simulink subsystem "rss_motor_model"  (R2023a)
settings: Solver=VariableStepAuto  StartTime=0.0  StopTime=10.0  RelTol=1e-3
undefined symbols (not defined in the file): Cdbl_indPhIndcPeakVal, Cdbl_psiPermMagFlxPeakVal, Cdbl_resPhRstnPeakVal, cstPermMagTempCoef, cstPhsRsntTempCoef, Gu16_indDaxIndc_C, Gu16_indQaxIndc_C, Gu16_psiPermMagFlx_C, Gu16_resPhRstn_C, Gu8_numPPNum_C, parAmbPermMagFlux_u16p22b0, parAmbPhsRsnt_u16p20b0, parDirIndc_u16p29b0, parGmrSensAngErrInpData, parGmrSensAngErrLktData, parMotRtrInrt, parMotTorsViscDamp, parPermMagTempCoef_s16p23b0, parPhsRsntTempCoef_s16p23b0, parPolePairNum_u8n0b0, parQdrtIndc_u16p29b0
libraries: mcbcontrolslib x4, MERMASS11MSEREF x3, eeTransforms x2, EMPSMDQ301MSEREF x2, lib_park_transform x2, EMPSMD3E01MSEREF x1, autolibpmsminterior x1, autolibsharedcoupling x1, simulink x1
settings Model: Creator=CAV2OFO  LastModifiedBy=xiaoqiang.yuan
settings SolverCC: AlgebraicLoopSolver=TrustRegion
settings OptimizationCC: ReuseModelBlockBuffer=off
settings DebuggingCC: UnconnectedInputMsg=warning  UnconnectedOutputMsg=warning  UnconnectedLineMsg=warning
settings ModelReferenceCC: EnableRefExpFcnMdlSchedulingChecks=on
settings RTWCC: DLArmComputeVersion=19.05

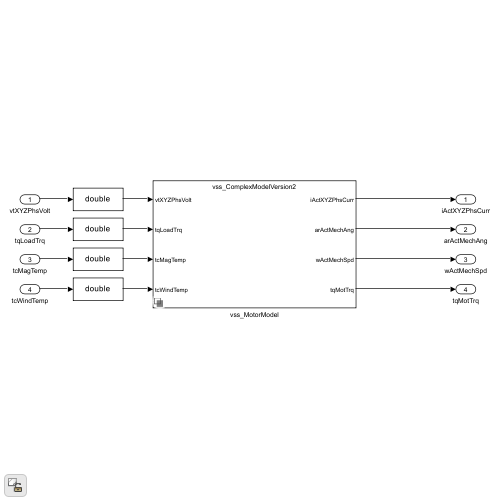
[thumbnail: Simulink's stored preview of the top-level diagram]
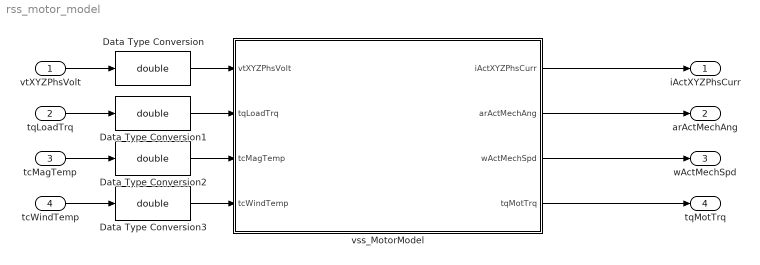
== system rss_motor_model ==
  vtXYZPhsVolt : Inport
  tqLoadTrq : Inport  Port=2
  tcMagTemp : Inport  Port=3
  tcWindTemp : Inport  Port=4
  Data Type Conversion{,1..3} (4 alike) : DataTypeConversion  OutDataTypeStr=double  SaturateOnIntegerOverflow=off  RndMeth=Floor
  vss_MotorModel : Subsystem  Variant=on  VariantControlMode=label  LabelModeActiveChoice=parCompMdlVrs2Lbl
  iActXYZPhsCurr : Outport
  arActMechAng : Outport  Port=2
  wActMechSpd : Outport  Port=3
  tqMotTrq : Outport  Port=4
  wires:
  vss_MotorModel/3(wActMechSpd) -> wActMechSpd/1
  vss_MotorModel/1(iActXYZPhsCurr) -> iActXYZPhsCurr/1
  vss_MotorModel/2(arActMechAng) -> arActMechAng/1
  tqLoadTrq/1 -> Data Type Conversion1/1
  vss_MotorModel/4(tqMotTrq) -> tqMotTrq/1
  vtXYZPhsVolt/1 -> Data Type Conversion/1
  tcMagTemp/1 -> Data Type Conversion2/1
  tcWindTemp/1 -> Data Type Conversion3/1
  Data Type Conversion/1 -> vss_MotorModel/1(vtXYZPhsVolt)
  Data Type Conversion1/1 -> vss_MotorModel/2(tqLoadTrq)
  Data Type Conversion3/1 -> vss_MotorModel/4(tcWindTemp)
  Data Type Conversion2/1 -> vss_MotorModel/3(tcMagTemp)

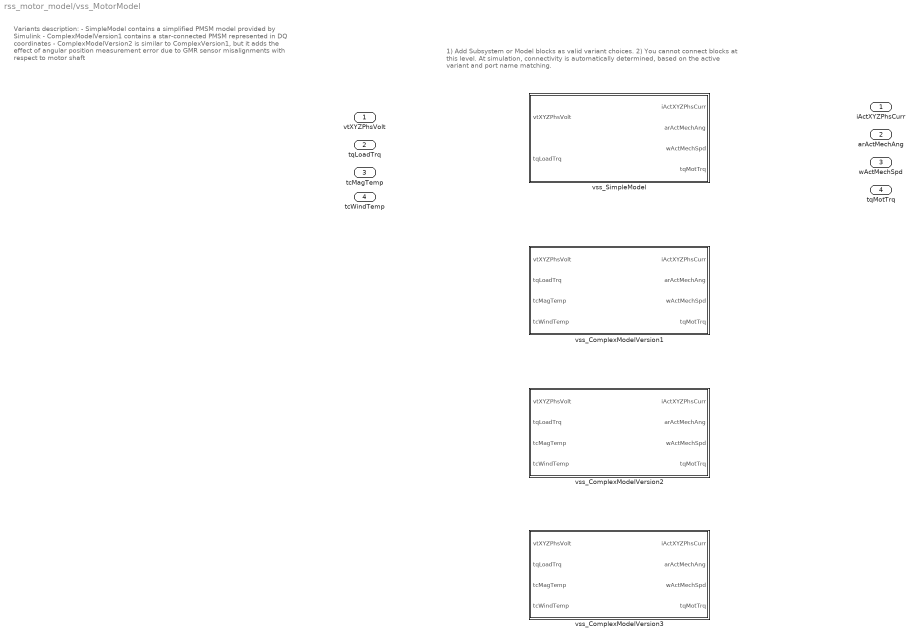
== system rss_motor_model/vss_MotorModel ==
  note: 1) Add Subsystem or Model blocks as valid variant choices.
      | 2) You cannot connect blocks at this level. At simulation, connectivity is automatically
      | determined, based on the active variant and port name matching.
  note: Variants description:
      | - SimpleModel contains a simplified PMSM model provided by Simulink
      | - ComplexModelVersion1 contains a star-connected PMSM represented
      | in DQ coordinates
      | - ComplexModelVersion2 is similar to ComplexVersion1, but it adds the
      | effect of angular position measurement error due to GMR sensor misalignments
      | with respect to motor shaft
  vtXYZPhsVolt : Inport
  tqLoadTrq : Inport  Port=2
  tcMagTemp : Inport  Port=3
  tcWindTemp : Inport  Port=4
  vss_ComplexModelVersion1 : Subsystem  VariantControl=parCompMdlVrs1Lbl
  vss_ComplexModelVersion2 : Subsystem  VariantControl=parCompMdlVrs2Lbl
  vss_ComplexModelVersion3 : Subsystem  VariantControl=Choice
  vss_SimpleModel : Subsystem  VariantControl=parSmplMdlLbl
  iActXYZPhsCurr : Outport
  arActMechAng : Outport  Port=2
  wActMechSpd : Outport  Port=3
  tqMotTrq : Outport  Port=4

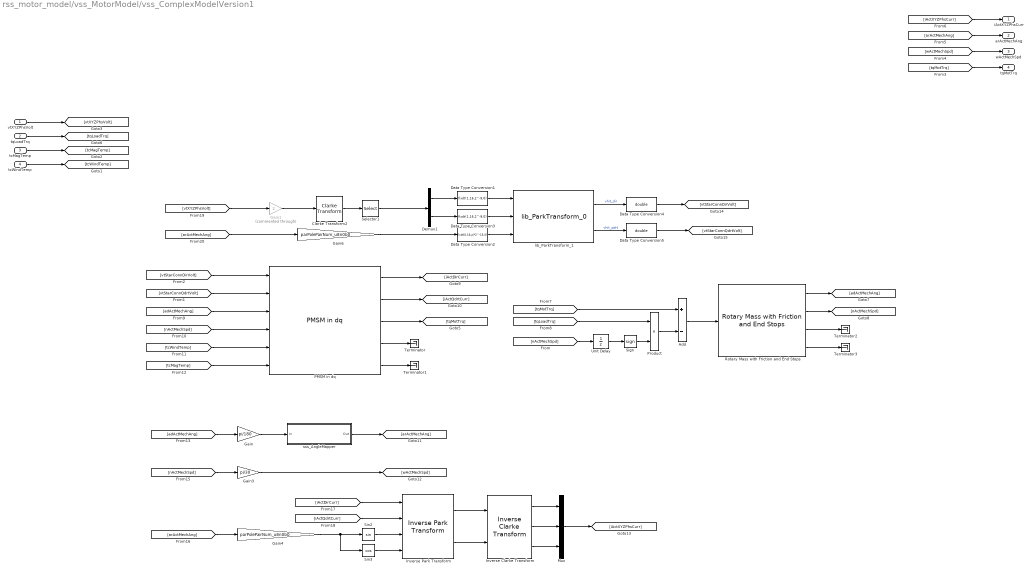
== system rss_motor_model/vss_MotorModel/vss_ComplexModelVersion1 ==
  vtXYZPhsVolt : Inport
  tqLoadTrq : Inport  Port=2
  tcMagTemp : Inport  Port=3
  tcWindTemp : Inport  Port=4
  Add : Sum  Inputs=+-
  Clarke Transform2 : eeTransforms/Clarke Transform  PowerInvariant=off
  Data Type Conversion1 : DataTypeConversion  OutDataTypeStr=fixdt(1,16,2^-9,0)  SaturateOnIntegerOverflow=off  RndMeth=Floor
  Data Type Conversion2 : DataTypeConversion  OutDataTypeStr=fixdt(0,16,pi*2^-15,0)  SaturateOnIntegerOverflow=off  RndMeth=Floor
  Data Type Conversion3 : DataTypeConversion  OutDataTypeStr=fixdt(1,16,2^-9,0)  SaturateOnIntegerOverflow=off  RndMeth=Floor
  Data Type Conversion4 : DataTypeConversion  OutDataTypeStr=double  SaturateOnIntegerOverflow=off  RndMeth=Floor
  Data Type Conversion5 : DataTypeConversion  OutDataTypeStr=double  SaturateOnIntegerOverflow=off  RndMeth=Floor
  Demux1 : Demux  Outputs=2
  Gain : Gain  Gain=pi/180
  Gain1 : Gain  Commented=through  Gain=2
  Gain3 : Gain  Gain=pi/30
  Gain4 : Gain  Gain=parPolePairNum_u8n0b0  OutDataTypeStr=double
  Gain6 : Gain  Gain=parPolePairNum_u8n0b0  OutDataTypeStr=double
  Inverse Clarke Transform : mcbcontrolslib/Inverse Clarke Transform  PhaseInput=Two inputs  EnPowerInv=off
  Inverse Park Transform : mcbcontrolslib/Inverse Park Transform  PhaseInput=Two inputs  AxisAlignment=D-axis  ThetaInput=Sine and Cosine electrical position  AngleInput=Per-unit  N_points=1024
  Mux : Mux  Inputs=3
  PMSM in dq : EMPSMDQ301MSEREF/PMSM in dq  Tag=EMPSMDQ301MSEREF  N=double(parPolePairNum_u8n0b0)  R20=double(parAmbPhsRsnt_u16p20b0)  Ld=double(parDirIndc_u16p29b0)  Lq=double(parQdrtIndc_u16p29b0)  Km20=double(parAmbPermMagFlux_u16p22b0)  Acog=0  Ncog=0  alpha=double(parPhsRsntTempCoef_s16p23b0)  alphamag=double(parPermMagTempCoef_s16p23b0)  xIdinit=0  xIqinit=0
      settings: AttributesFormatString=<%<Tag>>
  Product : Product
  Rotary Mass with Friction and End Stops : MERMASS11MSEREF/Rotary Mass with Friction and End Stops  Tag=MERMASS11MSEREF  J=double(parMotRtrInrt)  dvisc=double(parMotTorsViscDamp)*pi/30  frictionmode=no friction  epsn=0.001  tauinv=1000  TStick=1  TCoulomb=0.9  nStri=0.01  endstopmode=no end stop  phimin=-1e6  phimax=1e6  cstop=1e6  kimpact=0.5  phiinit=0  nRPMinit=0
      settings: AttributesFormatString=<%<Tag>>
  Selector1 : Selector  InputPortWidth=3  IndexOptions=Index vector (dialog)  Indices=[1 2]  OutputSizes=1
  Sign : Signum
  Sin2 : Trigonometry
  Sin3 : Trigonometry  Operator=cos
  Terminator{,1..3} (4 alike) : Terminator
  Unit Delay : UnitDelay  SampleTime=-1  HasFrameUpgradeWarning=on
  lib_ParkTransform_1 : lib_park_transform/lib_ParkTransform_0  VariantControl=ClarkTransf_MIL_flo  lb_parSelRotFrmeAxis=d-axis
  sss_AngleMapper : Subsystem
  iActXYZPhsCurr : Outport
  arActMechAng : Outport  Port=2
  wActMechSpd : Outport  Port=3
  tqMotTrq : Outport  Port=4
  wires:
  [arActMechAng] -> arActMechAng/1
  [tqLoadTrq] -> Product/1
  Unit Delay/1 -> Sign/1
  Sign/1 -> Product/2
  Product/1 -> Add/2
  [nActMechSpd] -> Unit Delay/1
  Gain1/1 -> Clarke Transform2/1
  Gain6/1 -> Data Type Conversion2/1
  Data Type Conversion5/1 -> [vtStarConnQdrtVolt]
  Clarke Transform2/1 -> Selector1/1
  lib_ParkTransform_1/1 -> Data Type Conversion4/1  "vhit_dir"
  [vtXYZPhsVolt] -> Gain1/1
  [arActMechAng] -> Gain6/1
  Data Type Conversion3/1 -> lib_ParkTransform_1/2
  Data Type Conversion1/1 -> lib_ParkTransform_1/1
  Data Type Conversion2/1 -> lib_ParkTransform_1/3
  Demux1/1 -> Data Type Conversion1/1
  Selector1/1 -> Demux1/1
  Demux1/2 -> Data Type Conversion3/1
  Data Type Conversion4/1 -> [vtStarConnDirVolt]
  lib_ParkTransform_1/2 -> Data Type Conversion5/1  "vhit_qdrt"
  Inverse Clarke Transform/3 -> Mux/3
  tcWindTemp/1 -> [tcWindTemp]
  [tcWindTemp] -> PMSM in dq/5
  Gain4/1 -> Sin2/1, Sin3/1
  Mux/1 -> [iActXYZPhsCurr]
  Inverse Park Transform/2 -> Inverse Clarke Transform/2
  Rotary Mass with Friction and End Stops/1 -> [adActMechAng]
  PMSM in dq/4 -> Terminator/1
  [arActMechAng] -> Gain4/1
  Rotary Mass with Friction and End Stops/4 -> Terminator3/1
  tqLoadTrq/1 -> [tqLoadTrq]
  [tqMotTrq] -> tqMotTrq/1
  vtXYZPhsVolt/1 -> [vtXYZPhsVolt]
  PMSM in dq/2 -> [iActQdrtCurr]
  [vtStarConnDirVolt] -> PMSM in dq/1
  [nActMechSpd] -> Gain3/1
  [iActDirCurr] -> Inverse Park Transform/1
  [iActQdrtCurr] -> Inverse Park Transform/2
  [adActMechAng] -> PMSM in dq/3
  Rotary Mass with Friction and End Stops/3 -> Terminator2/1
  [tcMagTemp] -> PMSM in dq/6
  Inverse Clarke Transform/1 -> Mux/1
  Inverse Park Transform/1 -> Inverse Clarke Transform/1
  PMSM in dq/5 -> Terminator1/1
  Gain3/1 -> [wActMechSpd]
  [tqMotTrq] -> Add/1
  [nActMechSpd] -> PMSM in dq/4
  sss_AngleMapper/1(Out) -> [arActMechAng]
  [vtStarConnQdrtVolt] -> PMSM in dq/2
  [wActMechSpd] -> wActMechSpd/1
  [iActXYZPhsCurr] -> iActXYZPhsCurr/1
  tcMagTemp/1 -> [tcMagTemp]
  PMSM in dq/3 -> [tqMotTrq]
  [adActMechAng] -> Gain/1
  Inverse Clarke Transform/2 -> Mux/2
  Add/1 -> Rotary Mass with Friction and End Stops/1
  Gain/1 -> sss_AngleMapper/1(In)
  Sin3/1 -> Inverse Park Transform/4
  Sin2/1 -> Inverse Park Transform/3
  PMSM in dq/1 -> [iActDirCurr]
  Rotary Mass with Friction and End Stops/2 -> [nActMechSpd]

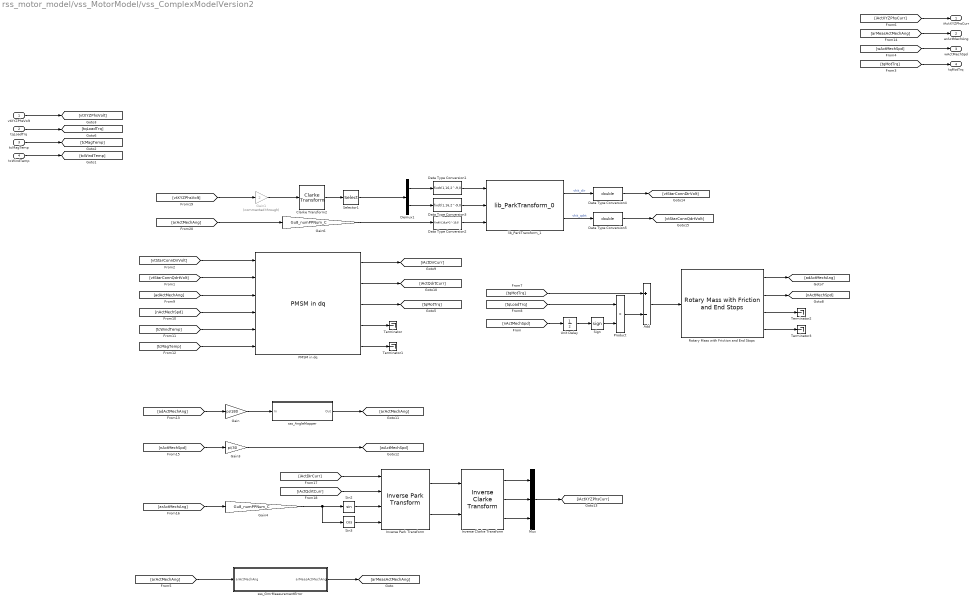
== system rss_motor_model/vss_MotorModel/vss_ComplexModelVersion2 ==
  vtXYZPhsVolt : Inport
  tqLoadTrq : Inport  Port=2
  tcMagTemp : Inport  Port=3
  tcWindTemp : Inport  Port=4
  Add : Sum  Inputs=+-
  Clarke Transform2 : eeTransforms/Clarke Transform  PowerInvariant=off
  Data Type Conversion1 : DataTypeConversion  OutDataTypeStr=fixdt(1,16,2^-9,0)  SaturateOnIntegerOverflow=off  RndMeth=Floor
  Data Type Conversion2 : DataTypeConversion  OutDataTypeStr=fixdt(0,16,pi*2^-15,0)  SaturateOnIntegerOverflow=off  RndMeth=Floor
  Data Type Conversion3 : DataTypeConversion  OutDataTypeStr=fixdt(1,16,2^-9,0)  SaturateOnIntegerOverflow=off  RndMeth=Floor
  Data Type Conversion4 : DataTypeConversion  OutDataTypeStr=double  SaturateOnIntegerOverflow=off  RndMeth=Floor
  Data Type Conversion5 : DataTypeConversion  OutDataTypeStr=double  SaturateOnIntegerOverflow=off  RndMeth=Floor
  Demux1 : Demux  Outputs=2
  Gain : Gain  Gain=pi/180
  Gain1 : Gain  Commented=through  Gain=2
  Gain3 : Gain  Gain=pi/30
  Gain4 : Gain  Gain=Gu8_numPPNum_C  OutDataTypeStr=double
  Gain6 : Gain  Gain=Gu8_numPPNum_C  OutDataTypeStr=double
  Inverse Clarke Transform : mcbcontrolslib/Inverse Clarke Transform
  Inverse Park Transform : mcbcontrolslib/Inverse Park Transform  AxisAlignment=D-axis
  Mux : Mux  Inputs=3
  PMSM in dq : EMPSMDQ301MSEREF/PMSM in dq  Tag=EMPSMDQ301MSEREF  N=double(Gu8_numPPNum_C)  R20=double(Gu16_resPhRstn_C*Cdbl_resPhRstnPeakVal)  Ld=double(Gu16_indDaxIndc_C*Cdbl_indPhIndcPeakVal)  Lq=double(Gu16_indQaxIndc_C*Cdbl_indPhIndcPeakVal)  Km20=double(Gu16_psiPermMagFlx_C*Cdbl_psiPermMagFlxPeakVal)  Acog=0  Ncog=0  alpha=double(cstPhsRsntTempCoef)  alphamag=double(cstPermMagTempCoef)  xIdinit=0  xIqinit=0
      settings: AttributesFormatString=<%<Tag>>
  Product : Product
  Rotary Mass with Friction and End Stops : MERMASS11MSEREF/Rotary Mass with Friction and End Stops  Tag=MERMASS11MSEREF  J=double(parMotRtrInrt)  dvisc=double(parMotTorsViscDamp)*pi/30  frictionmode=no friction  epsn=0.001  tauinv=1000  TStick=1  TCoulomb=0.9  nStri=0.01  endstopmode=no end stop  phimin=-1e6  phimax=1e6  cstop=1e6  kimpact=0.5  phiinit=rand*360  nRPMinit=0
      settings: AttributesFormatString=<%<Tag>>
  Selector1 : Selector  InputPortWidth=3  IndexOptions=Index vector (dialog)  Indices=[1 2]  OutputSizes=1
  Sign : Signum
  Sin2 : Trigonometry
  Sin3 : Trigonometry  Operator=cos
  Terminator{,1..3} (4 alike) : Terminator
  Unit Delay : UnitDelay  SampleTime=-1  HasFrameUpgradeWarning=on
  lib_ParkTransform_1 : lib_park_transform/lib_ParkTransform_0  VariantControl=ClarkTransf_MIL_flo  lb_parSelRotFrmeAxis=d-axis
  sss_AngleMapper : Subsystem
  sss_GmrMeasurementError : Subsystem
  iActXYZPhsCurr : Outport
  arActMechAng : Outport  Port=2
  wActMechSpd : Outport  Port=3
  tqMotTrq : Outport  Port=4
  wires:
  sss_GmrMeasurementError/1(arMeasActMechAng) -> [arMeasActMechAng]
  [arMeasActMechAng] -> arActMechAng/1
  [arActMechAng] -> sss_GmrMeasurementError/1(arActMechAng)
  [tqLoadTrq] -> Product/1
  Unit Delay/1 -> Sign/1
  Sign/1 -> Product/2
  Product/1 -> Add/2
  [nActMechSpd] -> Unit Delay/1
  Gain1/1 -> Clarke Transform2/1
  Gain6/1 -> Data Type Conversion2/1
  Data Type Conversion5/1 -> [vtStarConnQdrtVolt]
  Clarke Transform2/1 -> Selector1/1
  lib_ParkTransform_1/1 -> Data Type Conversion4/1  "vhit_dir"
  [vtXYZPhsVolt] -> Gain1/1
  [arActMechAng] -> Gain6/1
  Data Type Conversion3/1 -> lib_ParkTransform_1/2
  Data Type Conversion1/1 -> lib_ParkTransform_1/1
  Data Type Conversion2/1 -> lib_ParkTransform_1/3
  Demux1/1 -> Data Type Conversion1/1
  Selector1/1 -> Demux1/1
  Demux1/2 -> Data Type Conversion3/1
  Data Type Conversion4/1 -> [vtStarConnDirVolt]
  lib_ParkTransform_1/2 -> Data Type Conversion5/1  "vhit_qdrt"
  Inverse Clarke Transform/3 -> Mux/3
  tcWindTemp/1 -> [tcWindTemp]
  [tcWindTemp] -> PMSM in dq/5
  Gain4/1 -> Sin2/1, Sin3/1
  Mux/1 -> [iActXYZPhsCurr]
  Inverse Park Transform/2 -> Inverse Clarke Transform/2
  Rotary Mass with Friction and End Stops/1 -> [adActMechAng]
  PMSM in dq/4 -> Terminator/1
  [arActMechAng] -> Gain4/1
  Rotary Mass with Friction and End Stops/4 -> Terminator3/1
  tqLoadTrq/1 -> [tqLoadTrq]
  [tqMotTrq] -> tqMotTrq/1
  vtXYZPhsVolt/1 -> [vtXYZPhsVolt]
  PMSM in dq/2 -> [iActQdrtCurr]
  [vtStarConnDirVolt] -> PMSM in dq/1
  [nActMechSpd] -> Gain3/1
  [iActDirCurr] -> Inverse Park Transform/1
  [iActQdrtCurr] -> Inverse Park Transform/2
  [adActMechAng] -> PMSM in dq/3
  Rotary Mass with Friction and End Stops/3 -> Terminator2/1
  [tcMagTemp] -> PMSM in dq/6
  Inverse Clarke Transform/1 -> Mux/1
  Inverse Park Transform/1 -> Inverse Clarke Transform/1
  PMSM in dq/5 -> Terminator1/1
  Gain3/1 -> [wActMechSpd]
  [tqMotTrq] -> Add/1
  [nActMechSpd] -> PMSM in dq/4
  sss_AngleMapper/1(Out) -> [arActMechAng]
  [vtStarConnQdrtVolt] -> PMSM in dq/2
  [wActMechSpd] -> wActMechSpd/1
  [iActXYZPhsCurr] -> iActXYZPhsCurr/1
  tcMagTemp/1 -> [tcMagTemp]
  PMSM in dq/3 -> [tqMotTrq]
  [adActMechAng] -> Gain/1
  Inverse Clarke Transform/2 -> Mux/2
  Add/1 -> Rotary Mass with Friction and End Stops/1
  Gain/1 -> sss_AngleMapper/1(In)
  Sin3/1 -> Inverse Park Transform/4
  Sin2/1 -> Inverse Park Transform/3
  PMSM in dq/1 -> [iActDirCurr]
  Rotary Mass with Friction and End Stops/2 -> [nActMechSpd]

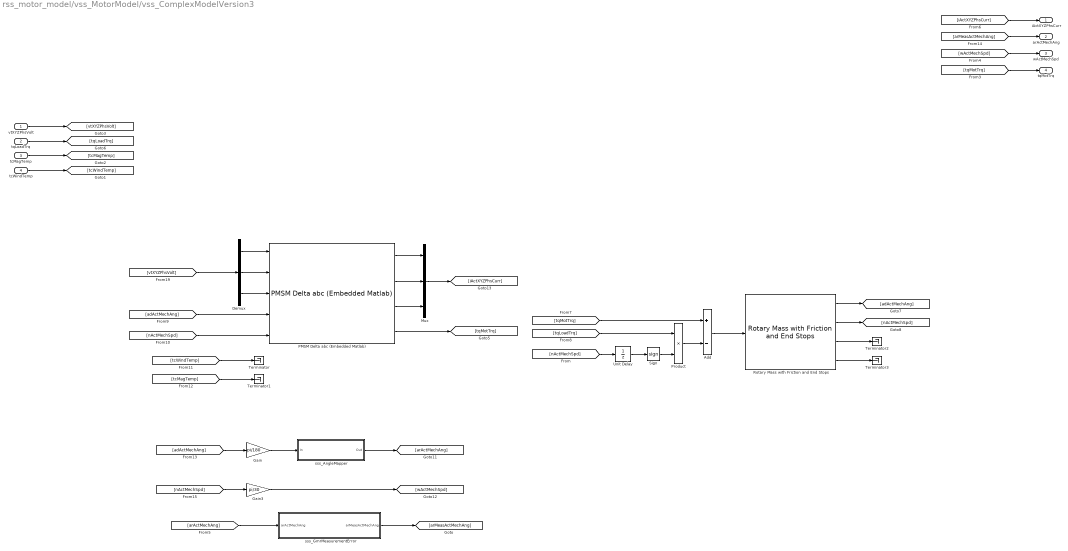
== system rss_motor_model/vss_MotorModel/vss_ComplexModelVersion3 ==
  vtXYZPhsVolt : Inport
  tqLoadTrq : Inport  Port=2
  tcMagTemp : Inport  Port=3
  tcWindTemp : Inport  Port=4
  Add : Sum  Inputs=+-
  Demux : Demux  Outputs=3
  Gain : Gain  Gain=pi/180
  Gain3 : Gain  Gain=pi/30
  Mux : Mux  Inputs=3
  PMSM Delta abc (Embedded Matlab) : EMPSMD3E01MSEREF/PMSM Delta abc (Embedded Matlab)  Tag=EMPSMD3E01MSEREF  N=double(parPolePairNum_u8n0b0)  r_m=double(parAmbPhsRsnt_u16p20b0)*3/2  l=[(double(parDirIndc_u16p29b0)+double(parQdrtIndc_u16p29b0))/2 0 (double(parDirIndc_u16p29b0)-double(parQdrtIndc_u16p29b0)) 0 0]*3/2  m=[0 0 0 0 0]  Km=double(parAmbPermMagFlux_u16p22b0)  a357=[0]  xIainit=0.0  xIbinit=0.0  xIcinit=0.0
      settings: AttributesFormatString=<%<Tag>>
  Product : Product
  Rotary Mass with Friction and End Stops : MERMASS11MSEREF/Rotary Mass with Friction and End Stops  Tag=MERMASS11MSEREF  J=double(parMotRtrInrt)  dvisc=double(parMotTorsViscDamp)*pi/30  frictionmode=no friction  epsn=0.001  tauinv=1000  TStick=1  TCoulomb=0.9  nStri=0.01  endstopmode=no end stop  phimin=-1e6  phimax=1e6  cstop=1e6  kimpact=0.5  phiinit=0  nRPMinit=0
      settings: AttributesFormatString=<%<Tag>>
  Sign : Signum
  Terminator{,1..3} (4 alike) : Terminator
  Unit Delay : UnitDelay  SampleTime=-1  HasFrameUpgradeWarning=on
  sss_AngleMapper : Subsystem
  sss_GmrMeasurementError : Subsystem
  iActXYZPhsCurr : Outport
  arActMechAng : Outport  Port=2
  wActMechSpd : Outport  Port=3
  tqMotTrq : Outport  Port=4
  wires:
  PMSM Delta abc (Embedded Matlab)/1 -> Mux/1
  PMSM Delta abc (Embedded Matlab)/2 -> Mux/2
  PMSM Delta abc (Embedded Matlab)/3 -> Mux/3
  Demux/3 -> PMSM Delta abc (Embedded Matlab)/3
  Demux/1 -> PMSM Delta abc (Embedded Matlab)/1
  Demux/2 -> PMSM Delta abc (Embedded Matlab)/2
  [adActMechAng] -> PMSM Delta abc (Embedded Matlab)/4
  [tqLoadTrq] -> Product/1
  Rotary Mass with Friction and End Stops/4 -> Terminator3/1
  sss_AngleMapper/1(Out) -> [arActMechAng]
  Add/1 -> Rotary Mass with Friction and End Stops/1
  [tcMagTemp] -> Terminator1/1
  vtXYZPhsVolt/1 -> [vtXYZPhsVolt]
  [nActMechSpd] -> Gain3/1
  [tcWindTemp] -> Terminator/1
  [tqMotTrq] -> tqMotTrq/1
  Rotary Mass with Friction and End Stops/1 -> [adActMechAng]
  Rotary Mass with Friction and End Stops/2 -> [nActMechSpd]
  tcMagTemp/1 -> [tcMagTemp]
  sss_GmrMeasurementError/1(arMeasActMechAng) -> [arMeasActMechAng]
  [vtXYZPhsVolt] -> Demux/1
  [iActXYZPhsCurr] -> iActXYZPhsCurr/1
  Unit Delay/1 -> Sign/1
  Gain3/1 -> [wActMechSpd]
  [arMeasActMechAng] -> arActMechAng/1
  Rotary Mass with Friction and End Stops/3 -> Terminator2/1
  [arActMechAng] -> sss_GmrMeasurementError/1(arActMechAng)
  Sign/1 -> Product/2
  Product/1 -> Add/2
  Mux/1 -> [iActXYZPhsCurr]
  tcWindTemp/1 -> [tcWindTemp]
  [nActMechSpd] -> Unit Delay/1
  [wActMechSpd] -> wActMechSpd/1
  Gain/1 -> sss_AngleMapper/1(In)
  [adActMechAng] -> Gain/1
  PMSM Delta abc (Embedded Matlab)/4 -> [tqMotTrq]
  [nActMechSpd] -> PMSM Delta abc (Embedded Matlab)/5
  tqLoadTrq/1 -> [tqLoadTrq]
  [tqMotTrq] -> Add/1

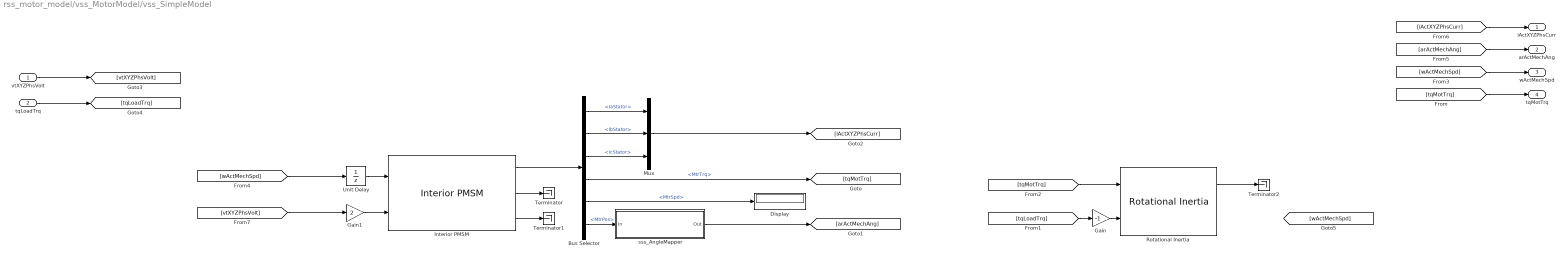
== system rss_motor_model/vss_MotorModel/vss_SimpleModel ==
  vtXYZPhsVolt : Inport
  tqLoadTrq : Inport  Port=2
  Bus Selector : BusSelector  OutputSignals=IaStator,IbStator,IcStator,MtrTrq,MtrSpd,MtrPos
  Display : Display
  Gain : Gain  Gain=-1
  Gain1 : Gain  Gain=2
  Interior PMSM : autolibpmsminterior/Interior PMSM  port_config=Speed  sim_type=Continuous  Ts=0.001  P=double(parPolePairNum_u8n0b0)  Rs=double(parAmbPhsRsnt_u16p20b0)  Ldq=double([parDirIndc_u16p29b0 parQdrtIndc_u16p29b0])  KConstText=Permanent flux linkage constant (lambda_pm):  lambda_pm=double(parAmbPermMagFlux_u16p22b0)  Ke=159.9771  mechanical=[0.002700,4.924e-4,0]  idq0=[0 0]  theta_init=0  omega_init=0  KConst=double(parAmbPermMagFlux_u16p22b0)  lambda_pm_calc=double(parAmbPermMagFlux_u16p22b0)  Kt=0.07  RefBlkName='autolibpmsminterior/Interior PMSM'  aMode=5
      settings: LibrarySourceBlock=mcblib/Electrical Systems/Motors/Interior PMSM
  Mux : Mux  Inputs=3
  Rotational Inertia : autolibsharedcoupling/Rotational Inertia  port_config=Simulink  extInfo=on  externJ=off  J=parMotRtrInrt  b=parMotTorsViscDamp  omega_o=0  blkID=0  aMode=2
      settings: LibrarySourceBlock=vdynlib/Powertrain/Drivetrain/Couplings/Rotational Inertia
  Terminator : Terminator
  Terminator1 : Terminator
  Terminator2 : Terminator
  Unit Delay : UnitDelay  SampleTime=-1  HasFrameUpgradeWarning=on
  sss_AngleMapper : Subsystem
  iActXYZPhsCurr : Outport
  arActMechAng : Outport  Port=2
  wActMechSpd : Outport  Port=3
  tqMotTrq : Outport  Port=4
  wires:
  Bus Selector/5 -> Display/1  "<MtrSpd>"
  [iActXYZPhsCurr] -> iActXYZPhsCurr/1
  Interior PMSM/2 -> Terminator/1
  Gain1/1 -> Interior PMSM/2
  Gain/1 -> Rotational Inertia/2
  Bus Selector/3 -> Mux/3  "<IcStator>"
  Unit Delay/1 -> Interior PMSM/1
  Interior PMSM/3 -> Terminator1/1
  Bus Selector/6 -> sss_AngleMapper/1(In)  "<MtrPos>"
  Interior PMSM/1 -> Bus Selector/1
  Bus Selector/2 -> Mux/2  "<IbStator>"
  Bus Selector/1 -> Mux/1  "<IaStator>"
  vtXYZPhsVolt/1 -> [vtXYZPhsVolt]
  [vtXYZPhsVolt] -> Gain1/1
  [tqMotTrq] -> tqMotTrq/1
  sss_AngleMapper/1(Out) -> [arActMechAng]
  Rotational Inertia/1 -> Terminator2/1
  Mux/1 -> [iActXYZPhsCurr]
  [tqMotTrq] -> Rotational Inertia/1
  [tqLoadTrq] -> Gain/1
  ? -> [wActMechSpd]
  Bus Selector/4 -> [tqMotTrq]  "<MtrTrq>"
  [arActMechAng] -> arActMechAng/1
  [wActMechSpd] -> wActMechSpd/1
  tqLoadTrq/1 -> [tqLoadTrq]
  [wActMechSpd] -> Unit Delay/1

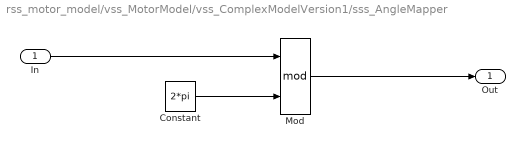
== system rss_motor_model/vss_MotorModel/vss_ComplexModelVersion1/sss_AngleMapper ==
  In : Inport
  Constant : Constant  Value=2*pi
  Mod : Math  Operator=mod
  Out : Outport
  wires:
  In/1 -> Mod/1
  Constant/1 -> Mod/2
  Mod/1 -> Out/1

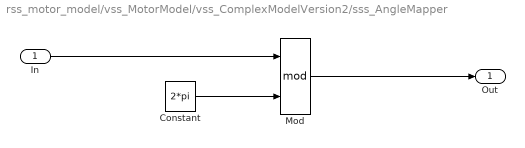
== system rss_motor_model/vss_MotorModel/vss_ComplexModelVersion2/sss_AngleMapper ==
  In : Inport
  Constant : Constant  Value=2*pi
  Mod : Math  Operator=mod
  Out : Outport
  wires:
  In/1 -> Mod/1
  Constant/1 -> Mod/2
  Mod/1 -> Out/1

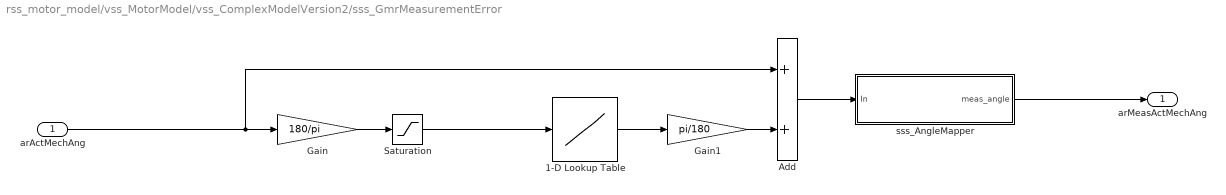
== system rss_motor_model/vss_MotorModel/vss_ComplexModelVersion2/sss_GmrMeasurementError ==
  arActMechAng : Inport
  1-D Lookup Table : Lookup_n-D  NumberOfTableDimensions=1  BreakpointsForDimension1=parGmrSensAngErrInpData  Table=parGmrSensAngErrLktData  InternalRulePriority=Speed  RndMeth=Simplest
  Add : Sum
  Gain : Gain  Gain=180/pi
  Gain1 : Gain  Gain=pi/180
  Saturation : Saturate  UpperLimit=360  LowerLimit=0
  sss_AngleMapper : Subsystem
  arMeasActMechAng : Outport
  wires:
  sss_AngleMapper/1(meas_angle) -> arMeasActMechAng/1
  Add/1 -> sss_AngleMapper/1(In)
  Gain1/1 -> Add/2
  1-D Lookup Table/1 -> Gain1/1
  Saturation/1 -> 1-D Lookup Table/1
  Gain/1 -> Saturation/1
  arActMechAng/1 -> Gain/1, Add/1

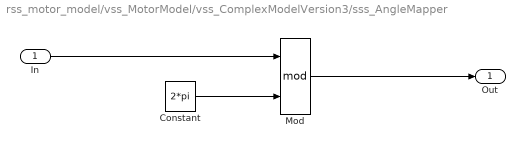
== system rss_motor_model/vss_MotorModel/vss_ComplexModelVersion3/sss_AngleMapper ==
  In : Inport
  Constant : Constant  Value=2*pi
  Mod : Math  Operator=mod
  Out : Outport
  wires:
  In/1 -> Mod/1
  Constant/1 -> Mod/2
  Mod/1 -> Out/1

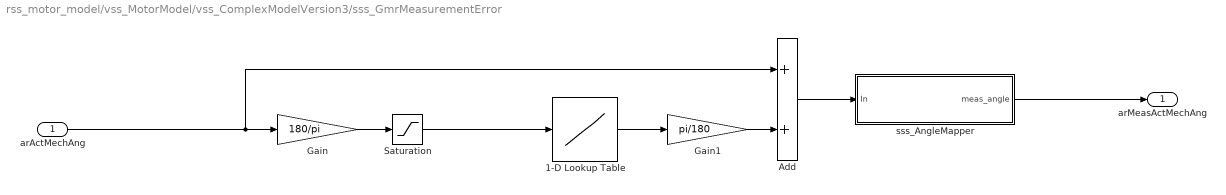
== system rss_motor_model/vss_MotorModel/vss_ComplexModelVersion3/sss_GmrMeasurementError ==
  arActMechAng : Inport
  1-D Lookup Table : Lookup_n-D  NumberOfTableDimensions=1  BreakpointsForDimension1=parGmrSensAngErrInpData  Table=parGmrSensAngErrLktData  InternalRulePriority=Speed  RndMeth=Simplest
  Add : Sum
  Gain : Gain  Gain=180/pi
  Gain1 : Gain  Gain=pi/180
  Saturation : Saturate  UpperLimit=360  LowerLimit=0
  sss_AngleMapper : Subsystem
  arMeasActMechAng : Outport
  wires:
  sss_AngleMapper/1(meas_angle) -> arMeasActMechAng/1
  Add/1 -> sss_AngleMapper/1(In)
  Gain1/1 -> Add/2
  1-D Lookup Table/1 -> Gain1/1
  Saturation/1 -> 1-D Lookup Table/1
  Gain/1 -> Saturation/1
  arActMechAng/1 -> Gain/1, Add/1

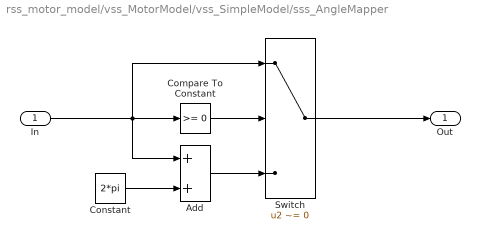
== system rss_motor_model/vss_MotorModel/vss_SimpleModel/sss_AngleMapper ==
  In : Inport
  Add : Sum
  Compare To Constant : simulink/Logic and Bit Operations/Compare To Constant  relop=>=  const=0  OutDataTypeStr=boolean
  Constant : Constant  Value=2*pi
  Switch : Switch  Criteria=u2 ~= 0  SaturateOnIntegerOverflow=off  InputSameDT=off
  Out : Outport
  wires:
  Switch/1 -> Out/1
  Constant/1 -> Add/2
  Add/1 -> Switch/3
  Compare To Constant/1 -> Switch/2
  In/1 -> Compare To Constant/1, Switch/1, Add/1

== system rss_motor_model/vss_MotorModel/vss_ComplexModelVersion2/sss_GmrMeasurementError/sss_AngleMapper ==
  In : Inport
  Constant : Constant  Value=2*pi
  Mod : Math  Operator=mod
  meas_angle : Outport
  wires:
  In/1 -> Mod/1
  Constant/1 -> Mod/2
  Mod/1 -> meas_angle/1

== system rss_motor_model/vss_MotorModel/vss_ComplexModelVersion3/sss_GmrMeasurementError/sss_AngleMapper ==
  In : Inport
  Constant : Constant  Value=2*pi
  Mod : Math  Operator=mod
  meas_angle : Outport
  wires:
  In/1 -> Mod/1
  Constant/1 -> Mod/2
  Mod/1 -> meas_angle/1
